simulink model "AddedMassTest"  (R2020a)
settings: Solver=VariableStepAuto  StartTime=0.0  StopTime=10.0  RelTol=1e-3
values from neighbouring files (symbols this model uses):
  eul = [0;pitch(i);0]*pi/180    [MonkMomentAnalysis.m]    (also in MunkMomentAnalysis.m = [0;pitch(jj);0]*pi/180)
  vFlow = [spd(j);0;0]    [MonkMomentAnalysis.m]    (also in MunkMomentAnalysis.m = [flwSpd(ii);0;0])
  vFlowGrad = zeros(3,6)    [MonkMomentAnalysis.m]
libraries: eulAng2RotMat_ul x1, addedMass_cl x1
settings Model: Creator=John Jr  LastModifiedBy=John Jr
settings DataIOCC: ReturnWorkspaceOutputs=off

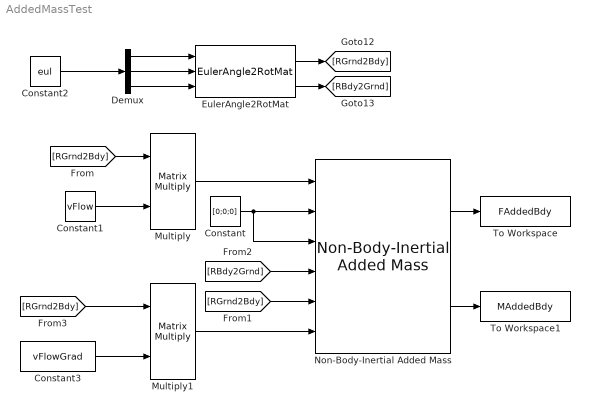
== system AddedMassTest ==
  Constant : Constant  Value=[0;0;0]
  Constant1 : Constant  Value=vFlow
  Constant2 : Constant  Value=eul
  Constant3 : Constant  Value=vFlowGrad
  Demux : Demux  Outputs=3
  EulerAngle2RotMat : eulAng2RotMat_ul/EulerAngle2RotMat  SystemSampleTime=-1  Latency=0  AutoFrameSizeCalculation=off
  Multiply : Product  Multiplication=Matrix(*)
  Multiply1 : Product  Multiplication=Matrix(*)
  Non-Body-Inertial Added Mass : addedMass_cl/Non-Body-Inertial Added Mass  MaMat=vhcl.Ma6x6_LE.Value  rB_LE=vhcl.rB_LE.Value  gradDist=vhcl.flowGradientDist.Value
  To Workspace : ToWorkspace  VariableName=FAddedBdy  SampleTime=-1
  To Workspace1 : ToWorkspace  VariableName=MAddedBdy  SampleTime=-1
  wires:
  Constant/1 -> Non-Body-Inertial Added Mass/3, Non-Body-Inertial Added Mass/2
  EulerAngle2RotMat/1 -> [RGrnd2Bdy]
  EulerAngle2RotMat/2 -> [RBdy2Grnd]
  Demux/1 -> EulerAngle2RotMat/1
  Demux/2 -> EulerAngle2RotMat/2
  Demux/3 -> EulerAngle2RotMat/3
  Constant2/1 -> Demux/1
  Multiply/1 -> Non-Body-Inertial Added Mass/1
  Constant1/1 -> Multiply/2
  [RGrnd2Bdy] -> Multiply/1
  [RGrnd2Bdy] -> Non-Body-Inertial Added Mass/5
  [RBdy2Grnd] -> Non-Body-Inertial Added Mass/4
  Multiply1/1 -> Non-Body-Inertial Added Mass/6
  Constant3/1 -> Multiply1/2
  [RGrnd2Bdy] -> Multiply1/1
  Non-Body-Inertial Added Mass/1 -> To Workspace/1
  Non-Body-Inertial Added Mass/2 -> To Workspace1/1
